simulink model "main"  (R2016b)
settings: Solver=FixedStepAuto  StartTime=0.0  StopTime=100  FixedStep=0.01  RelTol=1e-3
undefined symbols (not defined in the file): c, g, L, m, X, Y, Z
settings Model: Creator=Kumru  LastModifiedBy=Kumru

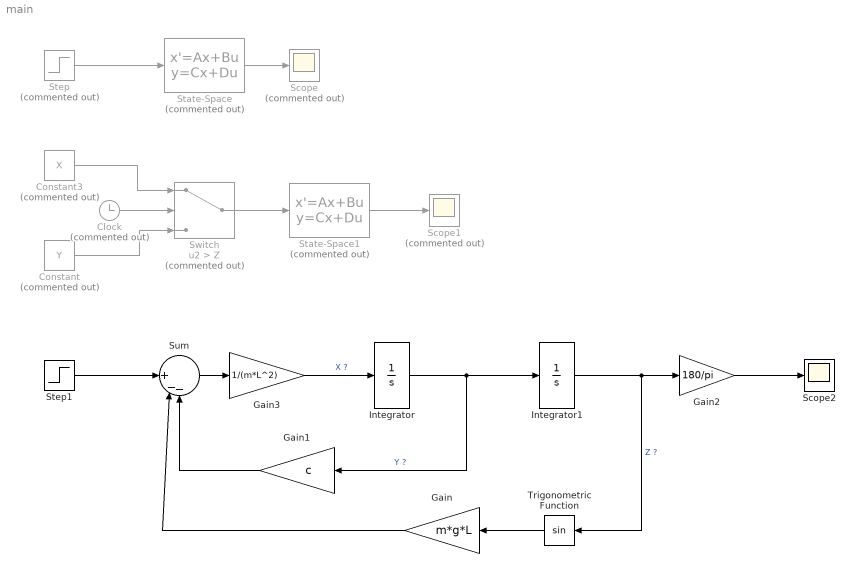
== system main ==
  Clock : Clock  Commented=on
  Constant : Constant  Commented=on  Value=Y
  Constant3 : Constant  Commented=on  Value=X
  Gain : Gain  Gain=m*g*L
  Gain1 : Gain  Gain=c
  Gain2 : Gain  Gain=180/pi
  Gain3 : Gain  Gain=1/(m*L^2)
  Integrator : Integrator
  Integrator1 : Integrator
  Scope : Scope  Commented=on
  Scope1 : Scope  Commented=on
  Scope2 : Scope
  State-Space : StateSpace  Commented=on  A=[0 1; -1 -2]  B=[0; 1]  C=[1 0]  D=0  X0=[0 0]
  State-Space1 : StateSpace  Commented=on  A=[0 1; -1 -1]  B=[0; 1]  C=[1 0]  D=0  X0=[0 0]
  Step : Step  Commented=on  Time=5  SampleTime=0
  Step1 : Step  Time=5  After=15  SampleTime=0
  Sum : Sum  Inputs=|||+|--
  Switch : Switch  Commented=on  Criteria=u2 > Threshold  Threshold=Z
  Trigonometric Function : Trigonometry
  wires:
  Step/1 -> State-Space/1
  State-Space/1 -> Scope/1
  Switch/1 -> State-Space1/1
  Constant/1 -> Switch/3
  Clock/1 -> Switch/2
  Constant3/1 -> Switch/1
  State-Space1/1 -> Scope1/1
  Trigonometric Function/1 -> Gain/1
  Integrator1/1 -> Trigonometric Function/1, Gain2/1  "Z ?"
  Integrator/1 -> Gain1/1, Integrator1/1  "Y ?"
  Sum/1 -> Gain3/1
  Gain1/1 -> Sum/3
  Gain/1 -> Sum/2
  Step1/1 -> Sum/1
  Gain2/1 -> Scope2/1
  Gain3/1 -> Integrator/1  "X ?"
